simulink model "Jose_Varela_mods3"  (Simulink 8.3)
settings: Solver=ode45  StartTime=0.0  StopTime=50  RelTol=1e-3
settings Model: Creator=FIE  LastModifiedBy=FIE
settings DataIOCC: SignalLoggingSaveFormat=Dataset
settings DebuggingCC: UnderspecifiedInitializationDetection=Simplified  StateNameClashWarn=none
settings RTWCC: GenCodeOnly=on
settings GRTTargetCC: CombineOutputUpdateFcns=on  GRTInterface=off

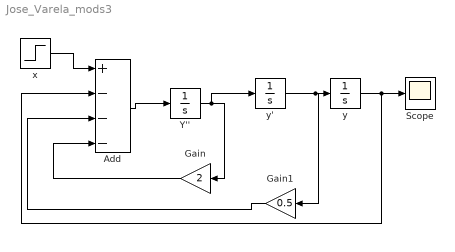
== system Jose_Varela_mods3 ==
  Add : Sum  Inputs=+---
  Gain : Gain  Gain=2
  Gain1 : Gain  Gain=0.5
  Scope : Scope
      settings: SaveName=Datos
  Y'' : Integrator
  x : Step  Time=0  SampleTime=0
  y : Integrator
  y' : Integrator
  wires:
  x/1 -> Add/1
  Add/1 -> Y''/1
  Y''/1 -> y'/1, Gain/1
  y'/1 -> Gain1/1, y/1
  Gain1/1 -> Add/3
  y/1 -> Scope/1, Add/2
  Gain/1 -> Add/4
